simulink model "modell"  (R2025b)
settings: Solver=FixedStepAuto  StartTime=0.0  StopTime=inf  FixedStep=0.1  RelTol=1e-3
libraries: simulink x1
settings Model: Creator=morten  LastModifiedBy=thomas-paulen
settings OptimizationCC: ReuseModelBlockBuffer=off
settings RTWCC: GPUComputeCapability=3.5

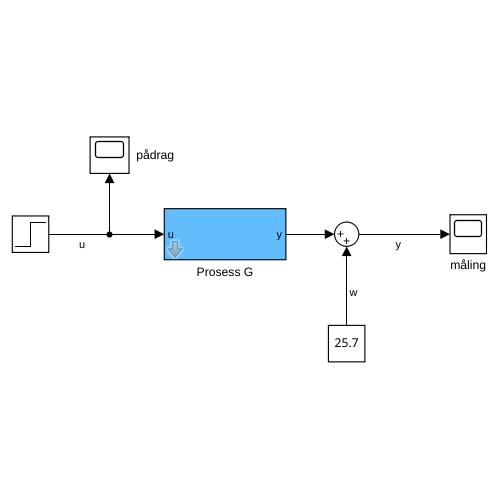
[thumbnail: Simulink's stored preview of the top-level diagram]
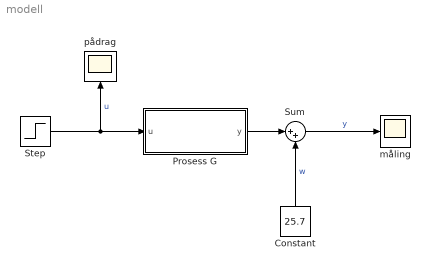
== system modell ==
  Constant : Constant  Value=25.7
  Prosess G : Subsystem
      mask DialogControl Control2 Prompt: Hjelpevideo:
      mask DialogControl Control3 Prompt: https://www.youtube.com/watch?v=dQw4w9WgXcQ
  Step : Step  Time=170  Before=1.5  After=120  SampleTime=0
  Sum : Sum  Inputs=|++
  måling : Scope
      settings: ActiveDisplayYMinimum=35.921786369490015  ActiveDisplayYMaximum=35.981202690435538
  pådrag : Scope
      settings: ActiveDisplayYMinimum=-179.791872398573  ActiveDisplayYMaximum=210.98993198759183
  wires:
  Step/1 -> pådrag/1, Prosess G/1(u)  "u"
  Prosess G/1(y) -> Sum/1
  Constant/1 -> Sum/2  "w"
  Sum/1 -> måling/1  "y"

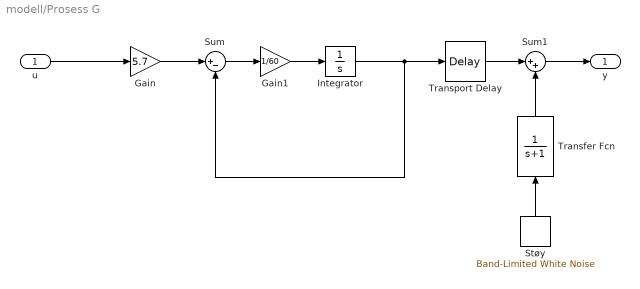
== system modell/Prosess G ==
  u : Inport
  Gain : Gain  Gain=5.7
  Gain1 : Gain  Gain=1/60
  Integrator : Integrator  InitialCondition=1.5*5.7
  Støy : simulink/Sources/Band-Limited White Noise  Cov=[0.0001]  Ts=0.1  seed=[23341]
  Sum : Sum  Inputs=|+-
  Sum1 : Sum  Inputs=|++
  Transfer Fcn : TransferFcn  Denominator=[1 1]
  Transport Delay : TransportDelay  DelayTime=4  InitialOutput=5.7*1.5
  y : Outport
  wires:
  u/1 -> Gain/1
  Sum/1 -> Gain1/1
  Gain1/1 -> Integrator/1
  Gain/1 -> Sum/1
  Integrator/1 -> Transport Delay/1, Sum/2
  Sum1/1 -> y/1
  Transport Delay/1 -> Sum1/1
  Støy/1 -> Transfer Fcn/1
  Transfer Fcn/1 -> Sum1/2
